simulink model "flying_walk_straight_kin_two_legs_RT_ready_2_1_show_"  (R2020a)
settings: Solver=ode15s  StartTime=0  StopTime=0.7  MaxStep=0.01  RelTol=1e-3  EnableMultiTasking=on
InitFcn:
  | servo_opacity=1;
values from neighbouring files (symbols this model uses):
  link0 = [1.0000         0         0    0.03891 ... (first row only)    [get_the_0angles_state_ext.m]
  link1 = [ -0.0000    0.0000   -1.0000    0.01001 ... (first row only)    [get_the_0angles_state_ext.m]
  link2 = [ 0.0000         0    1.0000    0.0555 ... (first row only)    [get_the_0angles_state_ext.m]
  link3 = [0.0000         0    1.0000   -0.0000 ... (first row only)    [get_the_0angles_state_ext.m]
  link4 = [1.0000         0         0   -0.03831 ... (first row only)    [get_the_0angles_state_ext.m]
  link5 = [1.0000         0         0   -0.05207 ... (first row only)    [get_the_0angles_state_ext.m]
  loop_initial_LL = [0 0 0 0 0 0]    [flying_control_file_remake.m]
  loop_initial_RL = [0 0 0 0 0 0]    [flying_control_file_remake.m]
  m_ll1 = 13.106e-3    (= 0.013106)    [masses.m]
  m_ll10 = 4.58 * 1e-3    (= 0.00458)    [masses.m]
  m_ll11 = 6.172 * 1e-3    (= 0.006172)    [masses.m]
  m_ll12 = 9.56 * 1e-3    (= 0.00956)    [masses.m]
  m_ll13 = 8.249 * 1e-3    (= 0.008249)    [masses.m]
  m_ll14 = 3.48 * 1e-3    (= 0.00348)    [masses.m]
  m_ll15 = 11.519 * 1e-3    (= 0.011519)    [masses.m]
  m_ll16 = 6.167 * 1e-3    (= 0.006167)    [masses.m]
  m_ll17 = 4.523 * 1e-3    (= 0.004523)    [masses.m]
  m_ll18 = 3.546 * 1e-3    (= 0.003546)    [masses.m]
  m_ll19 = 4.846 * 1e-3    (= 0.004846)    [masses.m]
  m_ll2 = 11.53e-3    (= 0.01153)    [masses.m]
  m_ll20 = 3.452 * 1e-3    (= 0.003452)    [masses.m]
  m_ll21 = 3.044 * 1e-3    (= 0.003044)    [masses.m]
  m_ll22 = 3.651 * 1e-3    (= 0.003651)    [masses.m]
  m_ll23 = 3.369 * 1e-3    (= 0.003369)    [masses.m]
  m_ll3 = 8.925 * 1e-3    (= 0.008925)    [masses.m]
  m_ll4 = 17.044 * 1e-3    (= 0.017044)    [masses.m]
  m_ll5 = 13.057 * 1e-3    (= 0.013057)    [masses.m]
  m_ll6 = 5.311 * 1e-3    (= 0.005311)    [masses.m]
  m_ll7 = 6.142 * 1e-3    (= 0.006142)    [masses.m]
  m_ll8 = 9.403 * 1e-3    (= 0.009403)    [masses.m]
  m_ll9 = 12.417 * 1e-3    (= 0.012417)    [masses.m]
  moi_ll1 = [2067.668 ... (first row only)    [masses.m]
  moi_ll10 = [1092.10 ... (first row only)    [masses.m]
  moi_ll10rl = [1092.10 ... (first row only)    [masses.m]
  moi_ll11 = [1426.607 ... (first row only)    [masses.m]
  moi_ll11rl = [1426.607 ... (first row only)    [masses.m]
  moi_ll12 = [3488.03 ... (first row only)    [masses.m]
  moi_ll12rl = [3488.03 ... (first row only)    [masses.m]
  moi_ll13 = [6377.723 ... (first row only)    [masses.m]
  moi_ll13rl = moi_ll13    [masses.m]
  moi_ll14 = [589.76 ... (first row only)    [masses.m]
  moi_ll14rl = moi_ll14    [masses.m]
  moi_ll15 = [1705.936 ... (first row only)    [masses.m]
  moi_ll15rl = moi_ll15    [masses.m]
  moi_ll16 = [2151.309 ... (first row only)    [masses.m]
  moi_ll16rl = moi_ll16    [masses.m]
  moi_ll17 = [953.485 ... (first row only)    [masses.m]
  moi_ll17rl = moi_ll17    [masses.m]
  moi_ll18 = [562.943 ... (first row only)    [masses.m]
  moi_ll18rl = moi_ll18    [masses.m]
  moi_ll19 = [3191.248 ... (first row only)    [masses.m]
  moi_ll19rl = moi_ll19    [masses.m]
  moi_ll1rl = [2067.668 ... (first row only)    [masses.m]
  moi_ll2 = [3083.915 ... (first row only)    [masses.m]
  moi_ll20 = [244.221 ... (first row only)    [masses.m]
  moi_ll20rl = moi_ll20    [masses.m]
  moi_ll21 = [140.841 ... (first row only)    [masses.m]
  moi_ll21rl = moi_ll21    [masses.m]
  moi_ll22 = [230.494 ... (first row only)    [masses.m]
  moi_ll22rl = moi_ll22    [masses.m]
  moi_ll23 = [157.913 ... (first row only)    [masses.m]
  moi_ll23rl = moi_ll23    [masses.m]
  moi_ll2rl = [3083.915 ... (first row only)    [masses.m]
  moi_ll3 = [2497.175 ... (first row only)    [masses.m]
  moi_ll3rl = [2497.175 ... (first row only)    [masses.m]
  moi_ll4 = [1.148E+04 ... (first row only)    [masses.m]
  moi_ll4rl = [1.148E+04 ... (first row only)    [masses.m]
  moi_ll5 = [9753.182 ... (first row only)    [masses.m]
  moi_ll5rl = [9753.182 ... (first row only)    [masses.m]
  moi_ll6 = [1161.983 ... (first row only)    [masses.m]
  moi_ll6rl = [1161.983 ... (first row only)    [masses.m]
  moi_ll7 = [1256.78 ... (first row only)    [masses.m]
  moi_ll7rl = [1256.78 ... (first row only)    [masses.m]
  moi_ll8 = [993.715 ... (first row only)    [masses.m]
  moi_ll8rl = [993.715 ... (first row only)    [masses.m]
  moi_ll9 = [2048.29 ... (first row only)    [masses.m]
  rlink0 = [1.0000         0         0    -0.03891 ... (first row only)    [get_the_0angles_state_ext.m]
  rlink1 = [ -0.0000    0.0000   1.0000    -0.01001 ... (first row only)    [get_the_0angles_state_ext.m]
  rlink2 = [ 1.0000         0    0.0000    0 ... (first row only)    [get_the_0angles_state_ext.m]
  rlink3 = [1.0000         0    0.0000   -0.014 ... (first row only)    [get_the_0angles_state_ext.m]
  rlink4 = [1.0000         0         0   0.0145 ... (first row only)    [get_the_0angles_state_ext.m]
  rlink5 = [0.0000         0         1   -0.0063 ... (first row only)    [get_the_0angles_state_ext.m]
  s = (1-T)./2    [evalcrdnd.m]
  servo_mass = 56.932e-3    (= 0.056932)    [masses.m]
undefined symbols (not defined in the file or in its folder): fir, MoI, PoI, rotation_fcn, translation_fcn, X, Y, Z
libraries: sm_lib x163, nesl_utility x13, simulink x12
(part 2 of 5)

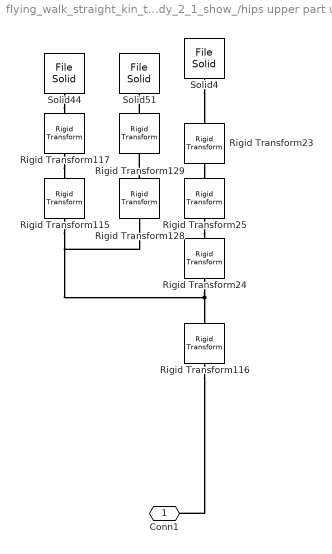
== system flying_walk_straight_kin_two_legs_RT_ready_2_1_show_/hips upper part visual ==
  Rigid Transform115 : sm_lib/Frames and Transforms/Rigid Transform  TranslationMethod=Cartesian  TranslationStandardOffset=0  TranslationLengthUnit=mm  TranslationStandardAxis=+Z  TranslationCartesianOffset="[33.03  29.492 -23.429]"  TranslationROffset=0  TranslationROffsetUnits=m  TranslationZOffset=0  TranslationZOffsetUnits=m  TranslationThetaOffset=0  TranslationThetaOffsetUnits=deg  RotationMethod=StandardAxis  RotationAngleUnits=deg  RotationStandardAxis=+Z  RotationAngle=180  RotationArbitraryAxis=[0 0 1]  FollAlignAxisA=+X  BaseAlignAxisA=+Y  FollAlignAxisB=+Y  BaseAlignAxisB=+Z  RotationSequenceAxes=FollowerAxes  RotationSequence=XYX  RotationSequenceAngles=[0 0 0]  RotationSequenceAnglesUnits=deg  RotationMatrix=[1 0 0; 0 1 0; 0 0 1]
  Rigid Transform116 : sm_lib/Frames and Transforms/Rigid Transform  TranslationMethod=Cartesian  TranslationStandardOffset=0  TranslationLengthUnit=mm  TranslationStandardAxis=+Z  TranslationCartesianOffset=[0 -11.24 0]  TranslationROffset=0  TranslationROffsetUnits=m  TranslationZOffset=0  TranslationZOffsetUnits=m  TranslationThetaOffset=0  TranslationThetaOffsetUnits=deg  RotationMethod=None  RotationAngleUnits=deg  RotationStandardAxis=+Z  RotationAngle=0.0  RotationArbitraryAxis=[0 0 1]  FollAlignAxisA=+X  BaseAlignAxisA=+Y  FollAlignAxisB=+Y  BaseAlignAxisB=+Z  RotationSequenceAxes=FollowerAxes  RotationSequence=XYX  RotationSequenceAngles=[0 0 0]  RotationSequenceAnglesUnits=deg  RotationMatrix=[1 0 0; 0 1 0; 0 0 1]
  Rigid Transform117 : sm_lib/Frames and Transforms/Rigid Transform  TranslationMethod=None  TranslationStandardOffset=0  TranslationLengthUnit=mm  TranslationStandardAxis=+Z  TranslationCartesianOffset="[33.03  29.492 -23.429]"  TranslationROffset=0  TranslationROffsetUnits=m  TranslationZOffset=0  TranslationZOffsetUnits=m  TranslationThetaOffset=0  TranslationThetaOffsetUnits=deg  RotationMethod=StandardAxis  RotationAngleUnits=deg  RotationStandardAxis=+Y  RotationAngle=35  RotationArbitraryAxis=[0 0 1]  FollAlignAxisA=+X  BaseAlignAxisA=+Y  FollAlignAxisB=+Y  BaseAlignAxisB=+Z  RotationSequenceAxes=FollowerAxes  RotationSequence=XYX  RotationSequenceAngles=[0 0 0]  RotationSequenceAnglesUnits=deg  RotationMatrix=[1 0 0; 0 1 0; 0 0 1]
  Rigid Transform128 : sm_lib/Frames and Transforms/Rigid Transform  TranslationMethod=Cartesian  TranslationStandardOffset=0  TranslationLengthUnit=mm  TranslationStandardAxis=+Z  TranslationCartesianOffset="[ -33.03  29.492 -23.492 ]"  TranslationROffset=0  TranslationROffsetUnits=m  TranslationZOffset=0  TranslationZOffsetUnits=m  TranslationThetaOffset=0  TranslationThetaOffsetUnits=deg  RotationMethod=StandardAxis  RotationAngleUnits=deg  RotationStandardAxis=+Z  RotationAngle=180  RotationArbitraryAxis=[0 0 1]  FollAlignAxisA=+X  BaseAlignAxisA=+Y  FollAlignAxisB=+Y  BaseAlignAxisB=+Z  RotationSequenceAxes=FollowerAxes  RotationSequence=XYX  RotationSequenceAngles=[0 0 0]  RotationSequenceAnglesUnits=deg  RotationMatrix=[1 0 0; 0 1 0; 0 0 1]
  Rigid Transform129 : sm_lib/Frames and Transforms/Rigid Transform  TranslationMethod=None  TranslationStandardOffset=0  TranslationLengthUnit=mm  TranslationStandardAxis=+Z  TranslationCartesianOffset="[33.03  29.492 -23.429]"  TranslationROffset=0  TranslationROffsetUnits=m  TranslationZOffset=0  TranslationZOffsetUnits=m  TranslationThetaOffset=0  TranslationThetaOffsetUnits=deg  RotationMethod=StandardAxis  RotationAngleUnits=deg  RotationStandardAxis=-Y  RotationAngle=35  RotationArbitraryAxis=[0 0 1]  FollAlignAxisA=+X  BaseAlignAxisA=+Y  FollAlignAxisB=+Y  BaseAlignAxisB=+Z  RotationSequenceAxes=FollowerAxes  RotationSequence=XYX  RotationSequenceAngles=[0 0 0]  RotationSequenceAnglesUnits=deg  RotationMatrix=[1 0 0; 0 1 0; 0 0 1]
  Rigid Transform23 : sm_lib/Frames and Transforms/Rigid Transform  TranslationMethod=Cartesian  TranslationStandardOffset=0  TranslationLengthUnit=mm  TranslationStandardAxis=+Z  TranslationCartesianOffset=[0.992 152.497 0]  TranslationROffset=0  TranslationROffsetUnits=m  TranslationZOffset=0  TranslationZOffsetUnits=m  TranslationThetaOffset=0  TranslationThetaOffsetUnits=deg  RotationMethod=None  RotationAngleUnits=deg  RotationStandardAxis=+Z  RotationAngle=0.0  RotationArbitraryAxis=[0 0 1]  FollAlignAxisA=+X  BaseAlignAxisA=+Y  FollAlignAxisB=+Y  BaseAlignAxisB=+Z  RotationSequenceAxes=FollowerAxes  RotationSequence=XYX  RotationSequenceAngles=[0 0 0]  RotationSequenceAnglesUnits=deg  RotationMatrix=[1 0 0; 0 1 0; 0 0 1]
  Rigid Transform24 : sm_lib/Frames and Transforms/Rigid Transform  TranslationMethod=None  TranslationStandardOffset=0  TranslationLengthUnit=mm  TranslationStandardAxis=+Z  TranslationCartesianOffset=[0.992 152.497 0]  TranslationROffset=0  TranslationROffsetUnits=m  TranslationZOffset=0  TranslationZOffsetUnits=m  TranslationThetaOffset=0  TranslationThetaOffsetUnits=deg  RotationMethod=StandardAxis  RotationAngleUnits=deg  RotationStandardAxis=+Y  RotationAngle=90  RotationArbitraryAxis=[0 0 1]  FollAlignAxisA=+X  BaseAlignAxisA=+Y  FollAlignAxisB=+Y  BaseAlignAxisB=+Z  RotationSequenceAxes=FollowerAxes  RotationSequence=XYX  RotationSequenceAngles=[0 0 0]  RotationSequenceAnglesUnits=deg  RotationMatrix=[1 0 0; 0 1 0; 0 0 1]
  Rigid Transform25 : sm_lib/Frames and Transforms/Rigid Transform  TranslationMethod=None  TranslationStandardOffset=0  TranslationLengthUnit=mm  TranslationStandardAxis=+Z  TranslationCartesianOffset=[0.992 152.497 0]  TranslationROffset=0  TranslationROffsetUnits=m  TranslationZOffset=0  TranslationZOffsetUnits=m  TranslationThetaOffset=0  TranslationThetaOffsetUnits=deg  RotationMethod=StandardAxis  RotationAngleUnits=deg  RotationStandardAxis=+Z  RotationAngle=90  RotationArbitraryAxis=[0 0 1]  FollAlignAxisA=+X  BaseAlignAxisA=+Y  FollAlignAxisB=+Y  BaseAlignAxisB=+Z  RotationSequenceAxes=FollowerAxes  RotationSequence=XYX  RotationSequenceAngles=[0 0 0]  RotationSequenceAnglesUnits=deg  RotationMatrix=[1 0 0; 0 1 0; 0 0 1]
  Solid4 : sm_lib/Body Elements/File Solid  ExtGeomFileName=..\stls\1 spine_3 servo_clamping_front_part_pelvis_v5.stl  UnitType=Custom  ExtGeomFileUnits=mm  StepReaderType=HEX  ExportConvexHullGeometry=off  InertiaType=Custom  Mass=0  MassUnits=kg  CenterOfMass=[0 0 0]  CenterOfMassUnits=m  MomentsOfInertia=[1 1 1]  MomentsOfInertiaUnits=kg*m^2  ProductsOfInertia=[0 0 0]  ProductsOfInertiaUnits=kg*m^2  BasedOnType=Density  Density=1000  DensityUnits=kg/(m^3)  DoExposeReferenceFrame=on  SerializedFrames=<Frames/>  GraphicType=FromGeometry  MarkerShape=Sphere  MarkerSize=10  MarkerSizeUnits=m  GraphicVisPropType=SimpleVisualProperties  GraphicDiffuseColor=[0.5 0.5 0.5]  GraphicSpecularColor=[0.5 0.5 0.5 1.0]  GraphicAmbientColor=[0.15 0.15 0.15 1.0]  GraphicEmissiveColor=[0.0 0.0 0.0 1.0]  GraphicShininess=75  GraphicOpacity=1.0
  Solid44 : sm_lib/Body Elements/File Solid  ExtGeomFileName=..\servo installing\servo1.stl  UnitType=Custom  ExtGeomFileUnits=mm  StepReaderType=HEX  ExportConvexHullGeometry=off  InertiaType=Custom  Mass=servo_mass  MassUnits=kg  CenterOfMass=servo_com  CenterOfMassUnits=m  MomentsOfInertia=servo_moi  MomentsOfInertiaUnits=kg*m^2  ProductsOfInertia=servo_poi  ProductsOfInertiaUnits=kg*m^2  BasedOnType=Density  Density=1000  DensityUnits=kg/(m^3)  DoExposeReferenceFrame=on  SerializedFrames=<Frames/>  GraphicType=FromGeometry  MarkerShape=Sphere  MarkerSize=10  MarkerSizeUnits=m  GraphicVisPropType=SimpleVisualProperties  GraphicDiffuseColor=[0.0 0.0 0.0]  GraphicSpecularColor=[0.5 0.5 0.5 1.0]  GraphicAmbientColor=[0.15 0.15 0.15 1.0]  GraphicEmissiveColor=[0.0 0.0 0.0 1.0]  GraphicShininess=75  GraphicOpacity=servo_opacity
  Solid51 : sm_lib/Body Elements/File Solid  ExtGeomFileName=..\servo installing\servo1.stl  UnitType=Custom  ExtGeomFileUnits=mm  StepReaderType=HEX  ExportConvexHullGeometry=off  InertiaType=Custom  Mass=servo_mass  MassUnits=kg  CenterOfMass=servo_com  CenterOfMassUnits=m  MomentsOfInertia=servo_moi  MomentsOfInertiaUnits=kg*m^2  ProductsOfInertia=servo_poi  ProductsOfInertiaUnits=kg*m^2  BasedOnType=Density  Density=1000  DensityUnits=kg/(m^3)  DoExposeReferenceFrame=on  SerializedFrames=<Frames/>  GraphicType=FromGeometry  MarkerShape=Sphere  MarkerSize=10  MarkerSizeUnits=m  GraphicVisPropType=SimpleVisualProperties  GraphicDiffuseColor=[0.0 0.0 0.0]  GraphicSpecularColor=[0.5 0.5 0.5 1.0]  GraphicAmbientColor=[0.15 0.15 0.15 1.0]  GraphicEmissiveColor=[0.0 0.0 0.0 1.0]  GraphicShininess=75  GraphicOpacity=servo_opacity
  Conn1 : PMIOPort  Side=Left
  connections:
  Rigid Transform25/RConn1 -- Rigid Transform24/LConn1
  Rigid Transform23/RConn1 -- Rigid Transform25/LConn1
  Solid44/RConn1 -- Rigid Transform117/RConn1
  Solid4/RConn1 -- Rigid Transform23/LConn1
  Rigid Transform24/RConn1 -- Rigid Transform116/RConn1 -- Rigid Transform128/LConn1 -- Rigid Transform115/LConn1
  Rigid Transform117/LConn1 -- Rigid Transform115/RConn1
  Rigid Transform129/RConn1 -- Solid51/RConn1
  Rigid Transform128/RConn1 -- Rigid Transform129/LConn1
  Rigid Transform116/LConn1 -- Conn1/RConn1

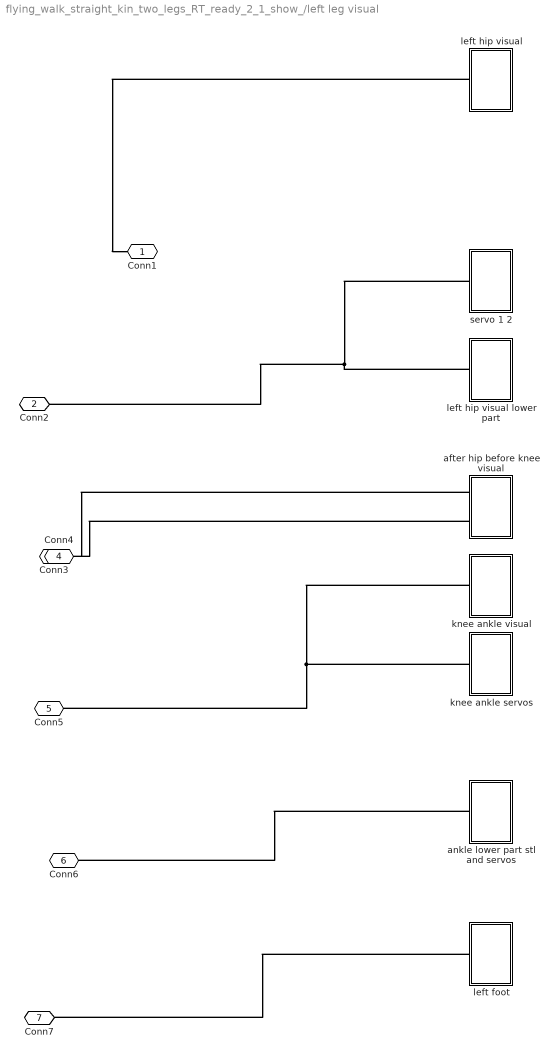
== system flying_walk_straight_kin_two_legs_RT_ready_2_1_show_/left leg visual ==
  after hip before knee visual : Subsystem
  ankle lower part stl and servos : Subsystem
  knee ankle servos : Subsystem
  knee ankle visual : Subsystem
  left foot : Subsystem
  left hip visual : Subsystem
  left hip visual lower part : Subsystem
  "servo 1 2 " : Subsystem
  Conn1 : PMIOPort  Side=Right
  Conn2 : PMIOPort  Port=2  Side=Left
  Conn3 : PMIOPort  Port=3  Side=Left
  Conn4 : PMIOPort  Port=4  Side=Left
  Conn5 : PMIOPort  Port=5  Side=Left
  Conn6 : PMIOPort  Port=6  Side=Left
  Conn7 : PMIOPort  Port=7  Side=Left
  connections:
  ankle lower part stl and servos/LConn1 -- Conn6/RConn1
  left hip visual/RConn1 -- Conn1/RConn1
  after hip before knee visual/LConn2 -- Conn4/RConn1
  knee ankle servos/LConn1 -- Conn5/RConn1 -- knee ankle visual/LConn1
  after hip before knee visual/LConn1 -- Conn3/RConn1
  "servo 1 2 "/LConn1 -- Conn2/RConn1 -- left hip visual lower part/LConn1
  left foot/LConn1 -- Conn7/RConn1
